simulink model "MicroFSMPCCLACPU1"  (R2024a)
settings: Solver=FixedStepAuto  StartTime=0.0  StopTime=Inf  RelTol=1e-3  EnableMultiTasking=on
values from neighbouring files (symbols this model uses):
  ar = single(round(1/10,3))    [Para_Motor_Micro.m]
  PI_params = mcb.internal.SetControllerParameters(pmsm,inverter,SI_System,T_pwm,Ts,Ts_speed)    [Para_Motor_Micro.m]
  Tabf = round(Tab',3)    [Para_Motor_Micro.m]
  target = mcb_SetProcessorDetails('F28379D',PWM_frequency)    [Para_Motor_Micro.m]
  Ts = T_pwm    (= 3e-05)    [Para_Motor_Micro.m]
  Ts_com = 2*1*Ts    (= 6e-05)    [Para_Motor_Micro.m]
undefined symbols (not defined in the file or in its folder): C28x, codertarget, CPU1, CPU2, Down, dyV, gmax, GPTRIP1SEL, GPTRIP2SEL, inverter, Ls, PWM_Counter_PeriodVel, R, Tab, Tv, Tvz, TZ1, TZ2, ud, Up
libraries: mcbcontrolslib x28, c2802xlib x18, c2837xDlib x13, dsparch4 x6, eeTransforms x5, slpidlib x4, mcbpositiondecoderlib x3, simulink x2, c2806xlib x1, spsabctoAlphaBetaZeroLib x1, c280xlib x1, c2000lib x1
(part 3 of 8)

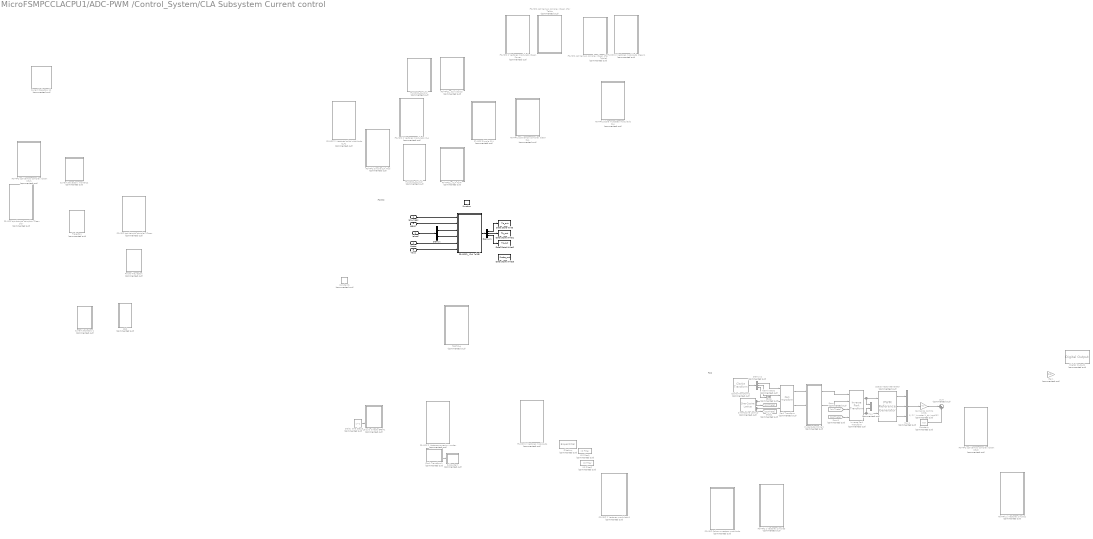
== system MicroFSMPCCLACPU1/ADC-PWM /Control_System/CLA Subsystem Current control ==
  note: FOC
  note: FSMPC
  Iab_meas : Inport
  Iabref : Inport  Port=2
  BEMF : Inport  Port=3
  Moder : Inport  Port=4
  Vbus : Inport  Port=5
  function : TriggerPort  TriggerType=function-call  VariantControl=(inherit)
  Calculo directo BFEM1 : MATLAB Function  Commented=on  TreatAsAtomicUnit=on
  Clark Transform1 : Subsystem  Commented=on
      settings: PortSchema="{\"entries\":[{\"content\":{\"sides\":[{\"content\":{\"connectorIds\":[\"In1\"]},\"type\":\"ConnectorPlacement.EquallySpacedRectSide\",\"uuid\":\"66940a32-98ed-4d42-b87c-a168e8060b1d\"},{\"content\":{\"connectorIds\":[\"Out1\",\"Out2\"],\"side\":\"RIGHT\"},\"type\":\"ConnectorPlacement.EquallySpacedRectSide\",\"uuid\":\"b045ffba-b3d8-4121-bbdc-9875b01ad1c0\"},{\"content\":{\"connectorIds\":[],\"side\":\"TOP\"},\"type\":\"ConnectorPlacement.EquallySpacedRectSide\",\"uuid\":\"4e19d047-7512-4d3b-a0ed-f9cfdeafce15\"},{\"content\":{\"connectorIds\":[\"In2\"],\"side\":\"BOTTOM\"},\"type\":\"ConnectorPlacement.EquallySpacedRectSide\",\"uuid\":\"62e76eb5-f8bd-4841-a5e0-53accc8eabe6\"}]},\"type\":\"ConnectorPlacement.EquallySpacedConnector\",\"uuid\":\"928147e2-84f8-479f-baed-93678fbc2e69\"}],\"packageUris\":[\"http://schema.mathworks.com/mf0/Connector/R2020b\"],\"version\":\"1.0\"}"
  Clarke Transform2 : eeTransforms/Clarke Transform  Commented=on  PowerInvariant=off
  Constant : Constant  Commented=on  Value=0.5  OutDataTypeStr=dataType  SampleTime=-1
  Constant1 : Constant  Commented=on  Value=[0,0,0]  OutDataTypeStr=single
  Current trajectory1 : MATLAB Function  Commented=on  TreatAsAtomicUnit=on
  Current trajectory12 : MATLAB Function  Commented=on  TreatAsAtomicUnit=on
  Current trayectory moder12 : MATLAB Function  Commented=on  TreatAsAtomicUnit=on
  Current_Controllers : Subsystem  Commented=on
  Data Store Write : DataStoreWrite  DataStoreName=Ta_out  IndexOptions=Index vector (dialog)  Indices=1  OutputSizes=1
  Data Store Write1 : DataStoreWrite  DataStoreName=Tb_out  IndexOptions=Index vector (dialog)  Indices=1  OutputSizes=1
  Data Store Write2 : DataStoreWrite  DataStoreName=Tc_out  IndexOptions=Index vector (dialog)  Indices=1  OutputSizes=1
  Data Store Write3 : DataStoreWrite  DataStoreName=Probe_out  IndexOptions=Index vector (dialog)  Indices=1  OutputSizes=1
  Delay One Step3 : Delay  Commented=on  DelayLength=1
  Demux : Demux  Outputs=2
  Demux1 : Demux  Outputs=3
  Demux2 : Demux  Commented=on  Outputs=3
  Digital Output1 : c2837xDlib/Digital Output  Commented=on  GPIO_Number=GPIO32~GPIO39  GPIO_Bit0=off  GPIO_BIT0_Toggle=on  GPIO_Bit1=off  GPIO_BIT1_Toggle=off  GPIO_Bit2=off  GPIO_BIT2_Toggle=off  GPIO_Bit3=off  GPIO_BIT3_Toggle=off  GPIO_Bit4=off  GPIO_BIT4_Toggle=off  GPIO_Bit5=off  GPIO_BIT5_Toggle=off  GPIO_Bit6=off  GPIO_BIT6_Toggle=off  GPIO_Bit7=on  GPIO_BIT7_Toggle=off
  FS-MPC 2 Vectores correcion moder : MATLAB Function  Commented=on  TreatAsAtomicUnit=on
  FS-MPC 2 Vectores modulado : MATLAB Function  Commented=on  TreatAsAtomicUnit=on
  FS-MPC 2 Vectores modulado CLA : MATLAB Function  Commented=on  TreatAsAtomicUnit=on
  FS-MPC 2 Vectores modulado Clean Power : MATLAB Function  Commented=on  TreatAsAtomicUnit=on
  FS-MPC 2 Vectores modulado Clean1 : MATLAB Function  Commented=on  TreatAsAtomicUnit=on
  FS-MPC 2 Vectores modulado1 : MATLAB Function  Commented=on  TreatAsAtomicUnit=on
  FS-MPC 2 Vectores simple2 : MATLAB Function  Commented=on  TreatAsAtomicUnit=on
  FS-MPC 2 Vectores simple3 : MATLAB Function  Commented=on  TreatAsAtomicUnit=on
  FS-MPC 2 Vectores solos modulado CLA1 : MATLAB Function  Commented=on  TreatAsAtomicUnit=on
  FS-MPC Simple CLA : MATLAB Function  Commented=on  TreatAsAtomicUnit=on
  FS-MPC Simple CLA Mod : MATLAB Function  Commented=on  TreatAsAtomicUnit=on
  FS-MPC Sobre muestreo modulado : MATLAB Function  Commented=on  TreatAsAtomicUnit=on
  FS-MPC Sobre muestreo modulado CLA : MATLAB Function  Commented=on  TreatAsAtomicUnit=on
  FS-MPC opt tiempo complex Clean : MATLAB Function  Commented=on  TreatAsAtomicUnit=on
  FS-MPC opt tiempo complex Clean 1for : MATLAB Function  Commented=on  TreatAsAtomicUnit=on
  FS-MPC opt tiempo complex Clean 1for Table : MATLAB Function  Commented=on  TreatAsAtomicUnit=on
  FS-MPC opt tiempo complex Clean 1for Table1 : MATLAB Function  Commented=on  TreatAsAtomicUnit=on
  FS-MPC opt tiempo complex Clean 1for1 : MATLAB Function  Commented=on  TreatAsAtomicUnit=on
  FS-MPC opt tiempo complex Clean 1for2 : MATLAB Function  Commented=on  TreatAsAtomicUnit=on
  FS-MPC opt tiempo complex Clean CLA : MATLAB Function  Commented=on  TreatAsAtomicUnit=on
  FS-MPC1_ CLA 10s(21) : MATLAB Function  Commented=on  TreatAsAtomicUnit=on
  "FS-MPC1_ CLA 4s(9) " : MATLAB Function  Commented=on  TreatAsAtomicUnit=on
  "FS-MPC1_ CLA 7s(15) " : MATLAB Function  TreatAsAtomicUnit=on
  FS-MPC2_CLA(10) : MATLAB Function  Commented=on  TreatAsAtomicUnit=on
  FS-MPC2_CLA(21) : MATLAB Function  Commented=on  TreatAsAtomicUnit=on
  Filterlow : dsparch4/Biquad Filter  Tag=BlockMethodSubSystem  Commented=on  FilterSource=Dialog parameters  CoeffSource=Specify via dialog  FilterObject=BQF  IIRFiltStruct=Direct form II  BiQuadCoeffs=[1 1 0 1 0.350634150167160374 0]  ScaleValues=[0.675317075083580187;1]  IC=0  ICnum=0  ICden=0  a0Flag=Warning  optimizeScaleValues=on  ScaleValueMode=Specify via input port (g)  InputProcessing=Columns as channels (frame based)  roundingMode=Floor  overflowMode=off  scaleValueFracLength=14  denProdOutputFracLength=30  denAccumFracLength=30  secondMemoryFracLength=15
  From : From  Commented=on  GotoTag=sinTheta
  From1 : From  Commented=on  GotoTag=cosTheta
  Gain : Gain  Commented=on  Gain=0.9  OutDataTypeStr=single
  Goto : Goto  Commented=on  GotoTag=sinTheta
  Goto1 : Goto  Commented=on  GotoTag=cosTheta
  IIR Filter1 : mcbcontrolslib/IIR Filter  Commented=on  VariantControl=Low Pass Filter  VariantSelect=Low-pass  FilterConstantInputType=Specify via dialog  Filter_constant=0.3  advancedSettings=off  Ts=5e-5  cutOff_freq=1364.1852
  IIR Filter2 : mcbcontrolslib/IIR Filter  Commented=on  VariantControl=Low Pass Filter  VariantSelect=Low-pass  FilterConstantInputType=Specify via dialog  Filter_constant=0.3  advancedSettings=off  Ts=5e-5  cutOff_freq=1364.1852
  Inverse Park Transform : mcbcontrolslib/Inverse Park Transform  Commented=on  PhaseInput=Two inputs  AxisAlignment=D-axis  ThetaInput=Sine and Cosine electrical position  AngleInput=Per-unit  N_points=1024
  Mux : Mux  Commented=on  Inputs=2
  Mux1 : Mux  Commented=on  Inputs=3
  Normalize [-0.5 to 0.5]1 : Gain  Commented=on  Gain=1/ (2 * inverter.V_dc / sqrt(3))  RndMeth=Simplest  OutDataTypeStr=Inherit: Same as input
  Park Transform : mcbcontrolslib/Park Transform  Commented=on  PhaseInput=Two inputs  AxisAlignment=D-axis  ThetaInput=Sine and Cosine electrical position  AngleInput=Per-unit  N_points=1024
  Power Trayectory : MATLAB Function  Commented=on  TreatAsAtomicUnit=on
  Sine-Cosine Lookup : mcbcontrolslib/Sine-Cosine Lookup  Commented=on  AngleInput=Radians  N_points=1024  DatatypeInput=Inherit from input  Datatype=single
  Space Vector Generator : mcbcontrolslib/PWM Reference Generator  Commented=on  inSignal=Valphabeta  modType=SVM: space vector modulation
  Subsystem : Subsystem  Commented=on
  Sum : Sum  Commented=on  Inputs=|++
  TESTCLA : MATLAB Function  Commented=on
  Terminator2 : Terminator  Commented=on
  Trajectory : MATLAB Function  Commented=on  TreatAsAtomicUnit=on
  stp2 : MATLAB Function  Commented=on  TreatAsAtomicUnit=on
  wires:
  Demux/1 -> "FS-MPC1_ CLA 7s(15) "/3(iAref)
  Clark Transform1/2(Fcemab) -> Subsystem/1(FCEM)
  Current_Controllers/1(Vd_ref) -> Inverse Park Transform/1
  Delay One Step3/1 -> Calculo directo BFEM1/3(Iant)
  Park Transform/2 -> Current_Controllers/2(Iq)
  From/1 -> Inverse Park Transform/3
  Demux/2 -> "FS-MPC1_ CLA 7s(15) "/4(iBref)
  From1/1 -> Inverse Park Transform/4
  Inverse Park Transform/1 -> Mux/1, Space Vector Generator/1
  Park Transform/1 -> Current_Controllers/1(Id)
  Normalize [-0.5 to 0.5]1/1 -> Sum/1
  Space Vector Generator/3 -> Mux1/3
  Current_Controllers/2(Vq_ref) -> Inverse Park Transform/2
  Clarke Transform2/1 -> Demux2/1
  Constant/1 -> Sum/2
  Demux2/1 -> Park Transform/1
  Iabref/1 -> Demux/1
  Mux1/1 -> Normalize [-0.5 to 0.5]1/1
  Space Vector Generator/2 -> Mux1/2
  Space Vector Generator/1 -> Mux1/1
  Demux2/3 -> Terminator2/1
  Moder/1 -> "FS-MPC1_ CLA 7s(15) "/5(mode)
  Demux2/2 -> Park Transform/2
  Sine-Cosine Lookup/2 -> Park Transform/4, Goto1/1
  Sine-Cosine Lookup/1 -> Goto/1, Park Transform/3
  Inverse Park Transform/2 -> Space Vector Generator/2, Mux/2
  Demux1/1 -> Data Store Write/1
  Demux1/2 -> Data Store Write1/1
  Demux1/3 -> Data Store Write2/1
  BEMF/1 -> "FS-MPC1_ CLA 7s(15) "/2(FEM)
  Vbus/1 -> "FS-MPC1_ CLA 7s(15) "/6(ud)
  "FS-MPC1_ CLA 7s(15) "/1(Gate) -> Demux1/1
  Iab_meas/1 -> "FS-MPC1_ CLA 7s(15) "/1(I)

== system MicroFSMPCCLACPU1/ADC-PWM /Control_System/Clark Transform Filter ==
  Iabc : Inport
  Clarke Transformation : Subsystem  InitFcn=tic2000lib_licenseCheck  mask(Clarke Transformation){}
      mask help: This block performs transformation of three-phase quantities into balanced two-phase quadrature quantities. All inputs and outputs are signed 32-bit fixed-point numbers with Q value between 1 and 29.
      mask Help: eval('linkfoundation.util.openBlockHelp(''c28xdmclibclarketransformation'',''ecoder'')');
      mask Display:
      | port_label('input',1,'As');
      | port_label('input',2,'Bs');
      | port_label('Output',1,'Alpha');
      | port_label('Output',2,'Beta');
      | text(0.5,0.15, 'Clarke', 'horizontalalignment','center');
  Demux : Demux  Outputs=3
  Mux1 : Mux  Inputs=2
  Iab : Outport
  wires:
  Iabc/1 -> Demux/1
  Clarke Transformation/1(Out1) -> Mux1/1
  Clarke Transformation/2(Out2) -> Mux1/2
  Demux/2 -> Clarke Transformation/2(Ib)
  Demux/1 -> Clarke Transformation/1(Ia)
  Mux1/1 -> Iab/1

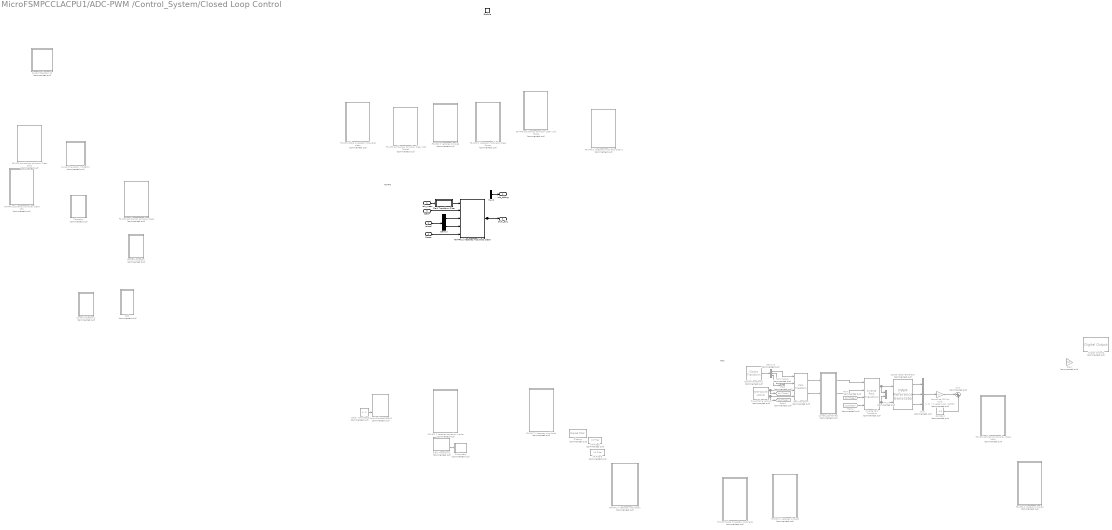
== system MicroFSMPCCLACPU1/ADC-PWM /Control_System/Closed Loop Control ==
  note: FSMPC
  note: FOC
  Iab_meas : Inport
  Iabref : Inport  Port=2
  BEMF : Inport  Port=3
  Moder : Inport  Port=4
  Enable : EnablePort  StatesWhenEnabling=reset
  Calculo directo BFEM1 : MATLAB Function  Commented=on  TreatAsAtomicUnit=on
  Clark Transform Filter : Subsystem
  Clark Transform1 : Subsystem  Commented=on
      settings: PortSchema="{\"entries\":[{\"content\":{\"sides\":[{\"content\":{\"connectorIds\":[\"In1\"]},\"type\":\"ConnectorPlacement.EquallySpacedRectSide\",\"uuid\":\"66940a32-98ed-4d42-b87c-a168e8060b1d\"},{\"content\":{\"connectorIds\":[\"Out1\",\"Out2\"],\"side\":\"RIGHT\"},\"type\":\"ConnectorPlacement.EquallySpacedRectSide\",\"uuid\":\"b045ffba-b3d8-4121-bbdc-9875b01ad1c0\"},{\"content\":{\"connectorIds\":[],\"side\":\"TOP\"},\"type\":\"ConnectorPlacement.EquallySpacedRectSide\",\"uuid\":\"4e19d047-7512-4d3b-a0ed-f9cfdeafce15\"},{\"content\":{\"connectorIds\":[\"In2\"],\"side\":\"BOTTOM\"},\"type\":\"ConnectorPlacement.EquallySpacedRectSide\",\"uuid\":\"62e76eb5-f8bd-4841-a5e0-53accc8eabe6\"}]},\"type\":\"ConnectorPlacement.EquallySpacedConnector\",\"uuid\":\"928147e2-84f8-479f-baed-93678fbc2e69\"}],\"packageUris\":[\"http://schema.mathworks.com/mf0/Connector/R2020b\"],\"version\":\"1.0\"}"
  Clarke Transform2 : eeTransforms/Clarke Transform  Commented=on  PowerInvariant=off
  Constant : Constant  Commented=on  Value=0.5  OutDataTypeStr=dataType  SampleTime=-1
  Current trajectory1 : MATLAB Function  Commented=on  TreatAsAtomicUnit=on
  Current trajectory12 : MATLAB Function  Commented=on  TreatAsAtomicUnit=on
  Current trayectory moder12 : MATLAB Function  Commented=on  TreatAsAtomicUnit=on
  Current_Controllers : Subsystem  Commented=on
  Delay One Step3 : Delay  Commented=on  DelayLength=1
  Demux : Demux  Outputs=2
  Demux2 : Demux  Commented=on  Outputs=3
  Digital Output1 : c2837xDlib/Digital Output  Commented=on  GPIO_Number=GPIO32~GPIO39  GPIO_Bit0=off  GPIO_BIT0_Toggle=on  GPIO_Bit1=off  GPIO_BIT1_Toggle=off  GPIO_Bit2=off  GPIO_BIT2_Toggle=off  GPIO_Bit3=off  GPIO_BIT3_Toggle=off  GPIO_Bit4=off  GPIO_BIT4_Toggle=off  GPIO_Bit5=off  GPIO_BIT5_Toggle=off  GPIO_Bit6=off  GPIO_BIT6_Toggle=off  GPIO_Bit7=on  GPIO_BIT7_Toggle=off
  FS-MPC 2 Vectores correcion moder : MATLAB Function  Commented=on  TreatAsAtomicUnit=on
  FS-MPC 2 Vectores modulado : MATLAB Function  Commented=on  TreatAsAtomicUnit=on
  FS-MPC 2 Vectores modulado Clean : MATLAB Function  TreatAsAtomicUnit=on
  FS-MPC 2 Vectores modulado Clean Power : MATLAB Function  Commented=on  TreatAsAtomicUnit=on
  FS-MPC 2 Vectores modulado Clean1 : MATLAB Function  Commented=on  TreatAsAtomicUnit=on
  FS-MPC 2 Vectores modulado1 : MATLAB Function  Commented=on  TreatAsAtomicUnit=on
  FS-MPC 2 Vectores simple1 : MATLAB Function  Commented=on  TreatAsAtomicUnit=on
  FS-MPC 2 Vectores simple2 : MATLAB Function  Commented=on  TreatAsAtomicUnit=on
  FS-MPC 2 Vectores simple3 : MATLAB Function  Commented=on  TreatAsAtomicUnit=on
  FS-MPC Sobre muestreo modulado : MATLAB Function  Commented=on  TreatAsAtomicUnit=on
  FS-MPC Sobre muestreo modulado clean : MATLAB Function  Commented=on  TreatAsAtomicUnit=on
  FS-MPC opt tiempo complex Clean : MATLAB Function  Commented=on  TreatAsAtomicUnit=on
  FS-MPC opt tiempo complex Clean 1for : MATLAB Function  Commented=on  TreatAsAtomicUnit=on
  FS-MPC opt tiempo complex Clean 1for Table : MATLAB Function  Commented=on  TreatAsAtomicUnit=on
  FS-MPC opt tiempo complex Clean 1for Table1 : MATLAB Function  Commented=on  TreatAsAtomicUnit=on
  FS-MPC opt tiempo complex Clean 1for1 : MATLAB Function  Commented=on  TreatAsAtomicUnit=on
  FS-MPC opt tiempo complex Clean 1for2 : MATLAB Function  Commented=on  TreatAsAtomicUnit=on
  Filterlow : dsparch4/Biquad Filter  Tag=BlockMethodSubSystem  Commented=on  FilterSource=Dialog parameters  CoeffSource=Specify via dialog  FilterObject=BQF  IIRFiltStruct=Direct form II  BiQuadCoeffs=[1 1 0 1 0.350634150167160374 0]  ScaleValues=[0.675317075083580187;1]  IC=0  ICnum=0  ICden=0  a0Flag=Warning  optimizeScaleValues=on  ScaleValueMode=Specify via input port (g)  InputProcessing=Columns as channels (frame based)  roundingMode=Floor  overflowMode=off  scaleValueFracLength=14  denProdOutputFracLength=30  denAccumFracLength=30  secondMemoryFracLength=15
  From : From  Commented=on  GotoTag=sinTheta
  From1 : From  Commented=on  GotoTag=cosTheta
  Gain : Gain  Commented=on  Gain=0.9  OutDataTypeStr=single
  Goto : Goto  Commented=on  GotoTag=sinTheta
  Goto1 : Goto  Commented=on  GotoTag=cosTheta
  IIR Filter1 : mcbcontrolslib/IIR Filter  Commented=on  VariantControl=Low Pass Filter  VariantSelect=Low-pass  FilterConstantInputType=Specify via dialog  Filter_constant=0.3  advancedSettings=off  Ts=5e-5  cutOff_freq=1364.1852
  IIR Filter2 : mcbcontrolslib/IIR Filter  Commented=on  VariantControl=Low Pass Filter  VariantSelect=Low-pass  FilterConstantInputType=Specify via dialog  Filter_constant=0.3  advancedSettings=off  Ts=5e-5  cutOff_freq=1364.1852
  Inverse Park Transform : mcbcontrolslib/Inverse Park Transform  Commented=on  PhaseInput=Two inputs  AxisAlignment=D-axis  ThetaInput=Sine and Cosine electrical position  AngleInput=Per-unit  N_points=1024
  Mux : Mux  Commented=on  Inputs=2
  Mux1 : Mux  Commented=on  Inputs=3
  Mux2 : Mux  Inputs=2
  Normalize [-0.5 to 0.5]1 : Gain  Commented=on  Gain=1/ (2 * inverter.V_dc / sqrt(3))  RndMeth=Simplest  OutDataTypeStr=Inherit: Same as input
  Park Transform : mcbcontrolslib/Park Transform  Commented=on  PhaseInput=Two inputs  AxisAlignment=D-axis  ThetaInput=Sine and Cosine electrical position  AngleInput=Per-unit  N_points=1024
  Power Trayectory : MATLAB Function  Commented=on  TreatAsAtomicUnit=on
  Sine-Cosine Lookup : mcbcontrolslib/Sine-Cosine Lookup  Commented=on  AngleInput=Radians  N_points=1024  DatatypeInput=Inherit from input  Datatype=single
  Space Vector Generator : mcbcontrolslib/PWM Reference Generator  Commented=on  inSignal=Valphabeta  modType=SVM: space vector modulation
  Subsystem : Subsystem  Commented=on
  Sum : Sum  Commented=on  Inputs=|++
  Terminator2 : Terminator  Commented=on
  Trajectory : MATLAB Function  Commented=on  TreatAsAtomicUnit=on
  stp2 : MATLAB Function  Commented=on  TreatAsAtomicUnit=on
  Idq_debug : Outport  VectorParamsAs1DForOutWhenUnconnected=off
  Duty_abc : Outport  Port=2  VectorParamsAs1DForOutWhenUnconnected=off
  wires:
  Park Transform/1 -> Current_Controllers/1(Id)
  Sine-Cosine Lookup/2 -> Park Transform/4, Goto1/1
  Sine-Cosine Lookup/1 -> Goto/1, Park Transform/3
  Demux2/2 -> Park Transform/2
  From1/1 -> Inverse Park Transform/4
  From/1 -> Inverse Park Transform/3
  Current_Controllers/1(Vd_ref) -> Inverse Park Transform/1
  Current_Controllers/2(Vq_ref) -> Inverse Park Transform/2
  Inverse Park Transform/1 -> Mux/1, Space Vector Generator/1
  Inverse Park Transform/2 -> Space Vector Generator/2, Mux/2
  Space Vector Generator/3 -> Mux1/3
  Space Vector Generator/2 -> Mux1/2
  Space Vector Generator/1 -> Mux1/1
  Normalize [-0.5 to 0.5]1/1 -> Sum/1
  Mux1/1 -> Normalize [-0.5 to 0.5]1/1
  Constant/1 -> Sum/2
  Park Transform/2 -> Current_Controllers/2(Iq)
  Demux2/3 -> Terminator2/1
  Clarke Transform2/1 -> Demux2/1
  Delay One Step3/1 -> Calculo directo BFEM1/3(Iant)
  Iab_meas/1 -> Clark Transform Filter/1(Iabc)
  Clark Transform Filter/1(Iab) -> FS-MPC 2 Vectores modulado Clean/1(I)
  Clark Transform1/2(Fcemab) -> Subsystem/1(FCEM)
  Mux2/1 -> Idq_debug/1
  Demux2/1 -> Park Transform/1
  Iabref/1 -> Demux/1
  BEMF/1 -> FS-MPC 2 Vectores modulado Clean/2(FEM)
  FS-MPC 2 Vectores modulado Clean/1(Gate) -> Duty_abc/1
  Demux/1 -> FS-MPC 2 Vectores modulado Clean/3(iAref)
  Demux/2 -> FS-MPC 2 Vectores modulado Clean/4(iBref)
  Moder/1 -> FS-MPC 2 Vectores modulado Clean/5(mode)

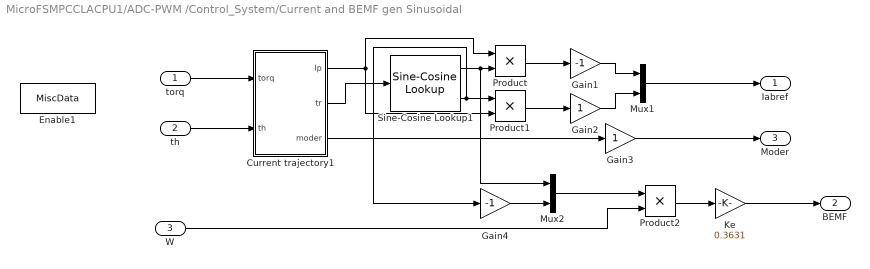
== system MicroFSMPCCLACPU1/ADC-PWM /Control_System/Current and BEMF gen Sinusoidal ==
  torq : Inport
  th : Inport  Port=2
  W : Inport  Port=3
  Current trajectory1 : MATLAB Function  TreatAsAtomicUnit=on
  Enable1 : DataStoreRead  DataStoreName=MiscData  IndexOptions=Index vector (dialog)  Indices=1  OutputSizes=1
  Gain1 : Gain  Gain=-1  OutDataTypeStr=single
  Gain2 : Gain  OutDataTypeStr=single
  Gain3 : Gain  OutDataTypeStr=single
  Gain4 : Gain  Gain=-1  OutDataTypeStr=single
  Ke : Gain  Gain=0.3631  OutDataTypeStr=single
  Mux1 : Mux  Inputs=2
  Mux2 : Mux  Inputs=2
  Product : Product  OutDataTypeStr=single
  Product1 : Product  OutDataTypeStr=single
  Product2 : Product  OutDataTypeStr=single
  Sine-Cosine Lookup1 : mcbcontrolslib/Sine-Cosine Lookup  AngleInput=Radians  N_points=1024  DatatypeInput=Specify via dialog  Datatype=single
  Iabref : Outport
  BEMF : Outport  Port=2
  Moder : Outport  Port=3
  wires:
  Current trajectory1/1(Ip) -> Product/1, Product1/2
  Mux2/1 -> Product2/1
  Sine-Cosine Lookup1/2 -> Gain4/1, Product1/1
  Product1/1 -> Gain2/1
  Product/1 -> Gain1/1
  torq/1 -> Current trajectory1/1(torq)
  W/1 -> Product2/2
  Product2/1 -> Ke/1
  Sine-Cosine Lookup1/1 -> Mux2/1, Product/2
  th/1 -> Current trajectory1/2(th)
  Current trajectory1/3(moder) -> Gain3/1
  Ke/1 -> BEMF/1
  Gain1/1 -> Mux1/1
  Gain2/1 -> Mux1/2
  Mux1/1 -> Iabref/1
  Gain3/1 -> Moder/1
  Gain4/1 -> Mux2/2
  Current trajectory1/2(tr) -> Sine-Cosine Lookup1/1

== system MicroFSMPCCLACPU1/ADC-PWM /Control_System/Current and BEMF gen Trapezoidal ==
  torq : Inport
  th : Inport  Port=2
  W : Inport  Port=3
  Current trajectory2 : MATLAB Function  TreatAsAtomicUnit=on
  Enable1 : DataStoreRead  DataStoreName=MiscData  IndexOptions=Index vector (dialog)  Indices=1  OutputSizes=1
  Mux : Mux  Inputs=2
  Iabref : Outport
  BEMF : Outport  Port=2
  Moder : Outport  Port=3
  wires:
  Current trajectory2/4(eab) -> BEMF/1
  th/1 -> Current trajectory2/2(th)
  torq/1 -> Current trajectory2/1(torq)
  W/1 -> Current trajectory2/3(w)
  Current trajectory2/2(Ib) -> Mux/2
  Current trajectory2/1(Ia) -> Mux/1
  Mux/1 -> Iabref/1
  Current trajectory2/3(moder) -> Moder/1

== system MicroFSMPCCLACPU1/ADC-PWM /Control_System/Te_calculation ==
  Iab : Inport
  Omega : Inport  Port=2
  FCEM : Inport  Port=3
  Add : Sum  Commented=on
  Demux : Demux  Commented=on  Outputs=2
  Demux1 : Demux  Commented=on  Outputs=2
  Divide : Product  Commented=on  Inputs=*/
  Gain : Gain  Commented=on  Gain=-1
  Product : Product  Commented=on
  Product1 : Product  Commented=on
  Te : Outport
  wires:
  Add/1 -> Divide/1
  Gain/1 -> Demux/1
  Demux/1 -> Product/1
  Demux1/2 -> Product1/2
  Product/1 -> Add/1
  Product1/1 -> Add/2
  FCEM/1 -> Gain/1
  Demux1/1 -> Product/2
  Omega/1 -> Divide/2
  Demux/2 -> Product1/1
  Iab/1 -> Demux1/1
  Divide/1 -> Te/1

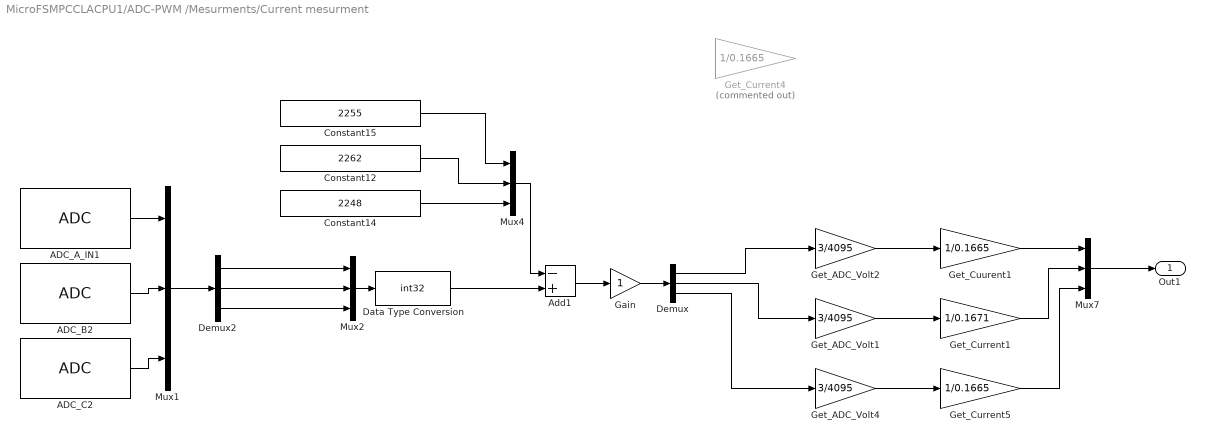
== system MicroFSMPCCLACPU1/ADC-PWM /Mesurments/Current mesurment ==
  ADC_A_IN1 : c2802xlib/ADC  blkParamProc=C2000_Type4  ADCModule=B  samplingMode=Single sample mode  ADCResolution=12-bit (Single-ended input)  useSOC1=SOC0  useSOC2=SOC0_SOC1  SOCAcquisitionWindow=15  SOCTriggerSource=ePWM1_ADCSOCA  SOCInterruptTrigger=No ADCINT  Ts=-1  dType=uint16  postInterrupt=off  interruptSel=ADCINT1  ADCINTContinuous=on  endma=off  chdma=1  conv1=ADCINA0  conv2=ADCINA0 and ADCINB0  conv1_Type4=ADCIN3  conv2_Type4=ADCIN0 and ADCIN1
  ADC_B2 : c2802xlib/ADC  blkParamProc=C2000_Type4  ADCModule=B  samplingMode=Single sample mode  ADCResolution=12-bit (Single-ended input)  useSOC1=SOC1  useSOC2=SOC0_SOC1  SOCAcquisitionWindow=15  SOCTriggerSource=ePWM1_ADCSOCA  SOCInterruptTrigger=No ADCINT  Ts=-1  dType=uint16  postInterrupt=off  interruptSel=ADCINT1  ADCINTContinuous=on  endma=off  chdma=1  conv1=ADCINA0  conv2=ADCINA0 and ADCINB0  conv1_Type4=ADCIN5  conv2_Type4=ADCIN0 and ADCIN1
  ADC_C2 : c2802xlib/ADC  blkParamProc=C2000_Type4  ADCModule=A  samplingMode=Single sample mode  ADCResolution=12-bit (Single-ended input)  useSOC1=SOC0  useSOC2=SOC0_SOC1  SOCAcquisitionWindow=15  SOCTriggerSource=ePWM1_ADCSOCA  SOCInterruptTrigger=No ADCINT  Ts=-1  dType=uint16  postInterrupt=on  interruptSel=ADCINT1  ADCINTContinuous=on  endma=off  chdma=1  conv1=ADCINA0  conv2=ADCINA0 and ADCINB0  conv1_Type4=ADCIN5  conv2_Type4=ADCIN0 and ADCIN1
  Add1 : Sum  Inputs=-+
  Constant12 : Constant  Value=2262  OutDataTypeStr=single
  Constant14 : Constant  Value=2248  OutDataTypeStr=single
  Constant15 : Constant  Value=2255  OutDataTypeStr=single
  Data Type Conversion : DataTypeConversion  OutDataTypeStr=int32  ConvertRealWorld=Stored Integer (SI)  RndMeth=Simplest  SaturateOnIntegerOverflow=off
  Demux : Demux  Outputs=3
  Demux2 : Demux  Outputs=3
  Gain : Gain  OutDataTypeStr=single
  Get_ADC_Volt1 : Gain  Gain=3/4095  OutDataTypeStr=single  RndMeth=Simplest
  Get_ADC_Volt2 : Gain  Gain=3/4095  OutDataTypeStr=single  RndMeth=Simplest
  Get_ADC_Volt4 : Gain  Gain=3/4095  OutDataTypeStr=single  RndMeth=Simplest
  Get_Current1 : Gain  Gain=1/0.1671  OutDataTypeStr=single  RndMeth=Simplest
  Get_Current4 : Gain  Commented=on  Gain=1/0.1665  OutDataTypeStr=single  RndMeth=Simplest
  Get_Current5 : Gain  Gain=1/0.1665  OutDataTypeStr=single  RndMeth=Simplest
  Get_Cuurent1 : Gain  Gain=1/0.1665  OutDataTypeStr=single  RndMeth=Simplest
  Mux{1..2,4,7} (4 alike) : Mux  Inputs=3
  Out1 : Outport
  wires:
  Data Type Conversion/1 -> Add1/2
  ADC_C2/1 -> Mux1/3
  Mux2/1 -> Data Type Conversion/1
  Demux2/2 -> Mux2/2
  Add1/1 -> Gain/1
  Demux2/3 -> Mux2/3
  Mux1/1 -> Demux2/1
  Mux4/1 -> Add1/1
  Demux/1 -> Get_ADC_Volt2/1
  ADC_B2/1 -> Mux1/2
  Constant12/1 -> Mux4/2
  Demux/2 -> Get_ADC_Volt1/1
  Get_ADC_Volt2/1 -> Get_Cuurent1/1
  ADC_A_IN1/1 -> Mux1/1
  Get_ADC_Volt4/1 -> Get_Current5/1
  Get_ADC_Volt1/1 -> Get_Current1/1
  Constant15/1 -> Mux4/1
  Demux/3 -> Get_ADC_Volt4/1
  Constant14/1 -> Mux4/3
  Demux2/1 -> Mux2/1
  Mux7/1 -> Out1/1
  Get_Cuurent1/1 -> Mux7/1
  Get_Current1/1 -> Mux7/2
  Get_Current5/1 -> Mux7/3
  Gain/1 -> Demux/1

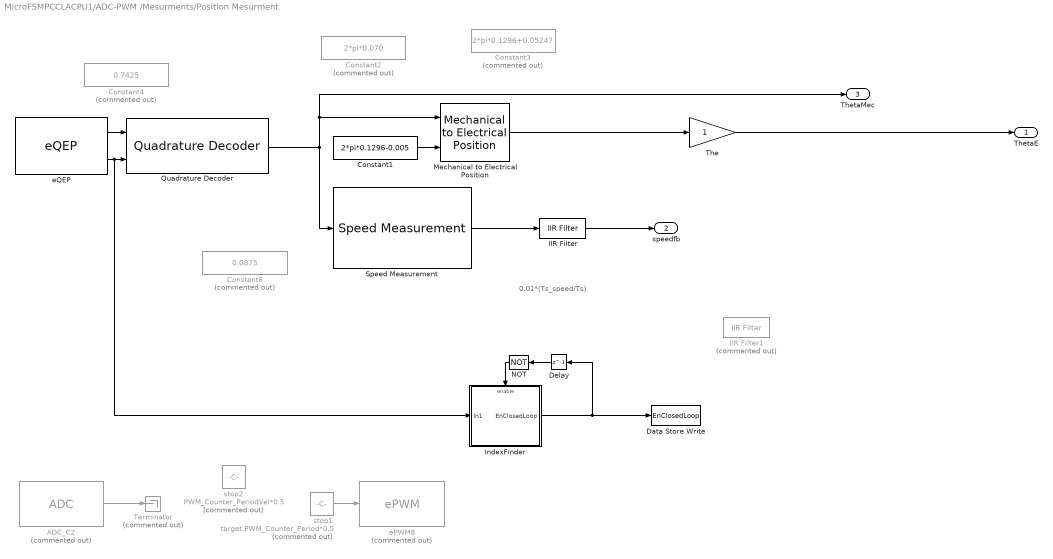
== system MicroFSMPCCLACPU1/ADC-PWM /Mesurments/Position Mesurment ==
  note: 0.01*(Ts_speed/Ts)
  ADC_C2 : c2802xlib/ADC  Commented=on  blkParamProc=C2000_Type4  ADCModule=C  samplingMode=Single sample mode  ADCResolution=12-bit (Single-ended input)  useSOC1=SOC5  useSOC2=SOC0_SOC1  SOCAcquisitionWindow=15  SOCTriggerSource=ePWM4_ADCSOCA  SOCInterruptTrigger=No ADCINT  Ts=-1  dType=uint16  postInterrupt=on  interruptSel=ADCINT1  ADCINTContinuous=on  endma=off  chdma=1  conv1=ADCINA0  conv2=ADCINA0 and ADCINB0  conv1_Type4=ADCIN0  conv2_Type4=ADCIN0 and ADCIN1
  Constant1 : Constant  Value=2*pi*0.1296-0.005  OutDataTypeStr=single
  Constant2 : Constant  Commented=on  Value=2*pi*0.070  OutDataTypeStr=single
  Constant3 : Constant  Commented=on  Value=2*pi*0.1296+0.05247  OutDataTypeStr=single
  Constant4 : Constant  Commented=on  Value=0.7425  OutDataTypeStr=single
  Constant6 : Constant  Commented=on  Value=0.0875  OutDataTypeStr=single
  Data Store Write : DataStoreWrite  DataStoreName=EnClosedLoop  IndexOptions=Index vector (dialog)  Indices=1  OutputSizes=1
  Delay : Delay  DelayLength=1
  IIR Filter : mcbcontrolslib/IIR Filter  VariantControl=Low Pass Filter  VariantSelect=Low-pass  FilterConstantInputType=Specify via dialog  Filter_constant=0.01  advancedSettings=off  Ts=10e-6  cutOff_freq=160.7626
  IIR Filter1 : mcbcontrolslib/IIR Filter  Commented=on  VariantControl=Low Pass Filter  VariantSelect=Low-pass  FilterConstantInputType=Specify via dialog  Filter_constant=0.0095  advancedSettings=off  Ts=10e-6  cutOff_freq=152.6473
  IndexFinder : Subsystem
  Mechanical to Electrical Position : mcbpositiondecoderlib/Mechanical to Electrical Position  PolePairsInputType=Specify via dialog  NrPP=4  selectedRange=Radians  MechOfstInputType=Input port  mechOffsetIn=0  maxAngleIn=2*pi  InputDataType=single  VariantSelect=floating-point
  NOT : Logic  Operator=NOT  AllPortsSameDT=off  OutDataTypeStr=boolean
  Quadrature Decoder : mcbpositiondecoderlib/Quadrature Decoder  EncoderSlitsPerRevolution=2048  EncoderCountsPerSlit=4  CounterSize=16 bits  ExternalIndexCount=on  PositionUnit=Radians  PositionDataType=single  ParameterInputType=off  CountsPerRevInverseDataType=single
  Speed Measurement : mcbpositiondecoderlib/Speed Measurement  PositionUnit=Radians  PositionScalingDatatype=uint32  SpeedCalculationMode=Time interval for speed calculation  SampleTimeAsync=Ts  MaximumApplicationSpeed=6000  SpeedResolution=5e-6  DelayLength=20  MaximumMeasurableSpeed=-0.98352  MeasurableSpeedResolution=7.6757e-12  SpeedUnit=Radians/Sec  PerUnitSpeed=PU_System.N_base  SpeedDataType=single
  Terminator : Terminator  Commented=on
  The : Gain  OutDataTypeStr=single  RndMeth=Simplest
  ePWM8 : c2802xlib/ePWM  Commented=on  PwmType=C2000_Type4  useModule=ePWM4  ePWMxLINKTBPRD=Not Linked  periodUnits=Clock cycles  timerSource=Specify via dialog  timerPeriod_clk=PWM_Counter_PeriodVel+1  timerPeriod_sec=0.0001  tbshadow=Counter equals to zero  countingMode=Up-Down  phaseActiveEnable=Disable  phaseDirection=Count down after sync  phaseActive=0  synchronizationEnable=off  dcaevt1Sync=off  dcbevt1Sync=off  synchronizationOption=Counter equals to zero (CTR=Zero)  dcbevt1SyncOut=off  dcaevt1SyncOut=off  cmpdSyncOut=off  cmpcSyncOut=off  cmpbSyncOut=off  zeroSyncOut=on  swfSyncOut=off  perSynchronizationOption=Counter equals to period (CTR=PRD)  clockPrescale=1  HSclockPrescale=1  enswap=off  ePWMxAStatus=on  ePWMxAactionLogic1=Do nothing  ePWMxAactionLogic2=Do nothing  ePWMxAactionLogic3=Clear  ePWMxAactionLogic4=Set  ePWMxAactionLogic5=Do nothing  ePWMxAactionLogic6=Do nothing  ePWMxACSFenable=off  ePWMxACSFvalue=Forcing disable  ePWMxASFreload=Zero  ePWMxBStatus=off  ePWMxBactionLogic1=Set  ePWMxBactionLogic2=Clear  ePWMxBactionLogic3=Do nothing  ePWMxBactionLogic4=Do nothing  ePWMxBactionLogic5=Clear  ePWMxBactionLogic6=Set  ePWMxBCSFenable=off  ePWMxBCSFvalue=Forcing disable  ePWMxBSFreload=Zero  ePWNxBOutWay=off  ePWMxLINKCMPA=Not Linked  CMPAUnits=Clock cycles  CMPASource=Input port  CMPAValue_per=50  CMPAValue_clk=floor(PWM_Counter_PeriodVel/2+1)  enCMPAshadow=Counter equals to zero (CTR=Zero)  ePWMxLINKCMPB=Not Linked  CMPBUnits=Clock cycles  CMPBSource=Specify via dialog  CMPBValue_per=50  CMPBValue_clk=floor(PWM_Counter_PeriodVel/2+1)  enCMPBshadow=Counter equals to zero (CTR=Zero)  ePWMxLINKCMPC=Not Linked  CMPCUnits=Clock cycles  CMPCSource=Specify via dialog  CMPCValue_per=50  CMPCValue_clk=32000  enCMPCshadow=Counter equals to zero (CTR=Zero)  ePWMxLINKCMPD=Not Linked  CMPDUnits=Clock cycles  CMPDSource=Specify via dialog  CMPDValue_per=50  CMPDValue_clk=32000  enCMPDshadow=Counter equals to zero (CTR=Zero)  enableDBePWMxA=on  enableDBePWMxB=on  enhalfcycle=off  DBpolarity=Active high complementary (AHC)  DBedgeDelay=Positive  DBSource_ePWMxA=ePWMxA  DBSource_ePWMxB=ePWMxA  DBPeriodUnits=Clock cycles  DBperiodSource=Specify via dialog  REDperiod=15  FEDperiod=15  REDperiod_sec=0  FEDperiod_sec=0  LoadModeDBRED=Immediate without using shadow  LoadModeDBFED=Immediate without using shadow  adcstartModuleA=on  adcrequestEventA=First event  adcstartEventA=Digital Compare Module A Event 1 start of conversion (DCAEVT1.soc)  adcstartEventA_type2=Counter equals to period (CTR=PRD)  adcstartModuleB=off  adcrequestEventB=First event  adcstartEventB=Counter equals to zero (CTR=Zero)  adcstartEventB_type2=Counter equals to zero (CTR=Zero)  intEn=off  intPrd=First event  intSel=Counter equals to zero (CTR=Zero)  intSel_type2=Counter equals to zero (CTR=Zero)  hrpe=off  enHRPWM=off  HRPWM_LoadMode=Counter equals to period (CTR=PRD)  HRPWM_CTLMode=Duty or Period control mode  HRPWM_EDGMode=Both edge  hrpeb=off  enHRPWMB=off  HRPWM_LoadModeB=Counter equals to zero (CTR=ZERO)  HRPWM_CTLModeB=Duty or Period control mode  HRPWM_EDGModeB=Both edge  enHRDBRED=off  enHRDBFED=off  enSFO=on  enautoconv=on  chopperEnable=off  chopperFrequency=1  chopperFirstwidth=1  chopperDuty=12.5%  tripZonesource=Specify via dialog  tzselOSHT1=off  tzselOSHT2=off  tzselOSHT3=off  tzselOSHT4=off  tzselOSHT5=off  tzselOSHT6=off  tzselOSHDCAEV1=off  tzselOSHDCBEV1=off  tzselCBC1=off  tzselCBC2=off  tzselCBC3=off  tzselCBC4=off  tzselCBC5=off  tzselCBC6=off  tzselCBCDCAEV2=off  tzselCBCDCBEV2=off  enTzOstIntr=off  enTzCbcIntr=off  enTzDCAEVT1Intr=off  enTzDCAEVT2Intr=off  enTzDCBEVT1Intr=off  enTzDCBEVT2Intr=off  tzclrCBCLatch=Counter equals to zero (CTR=Zero)  ePWMxAforced=No action  ePWMxBforced=No action  DCAEVT1forced=No action  DCBEVT1forced=No action  DCAEVT2forced=No action  DCBEVT2forced=No action  dcah=Trip Zone 1 input (TZ1)  dcal=Trip Zone 2 input (TZ2)  dcbh=Trip Zone 1 input (TZ1)  dcbl=Trip Zone 2 input (TZ2)  dcah_type2=GPTRIP1SEL/(TZ1)  dcal_type2=GPTRIP2SEL/(TZ2)  dcbh_type2=GPTRIP1SEL/(TZ1)  dcbl_type2=GPTRIP2SEL/(TZ2)  gendcaevt1=Event disabled  gendcaevt2=Event disabled  gendcbevt1=Event disabled  gendcbevt2=Event disabled  dcaevt1src=DCAEVT1 with sync  dcaevt2src=DCAEVT2 with sync  dcbevt1src=DCBEVT1 with sync  dcbevt2src=DCBEVT2 with sync  pulsesel=Counter equals to zero (CTR=Zero)  blankinv=off  blankoffset=0  blankwidth=0  evsrcsel=Filtered version of DCAEVT1 (DCAEVT1FILT)  encape=off
  eQEP : c280xlib/eQEP  useModule=eQEP1  pcInputmode=Quadrature-count  externalClockrate=2x resolution: Count the rising/falling edge  swapPolarityselection=Counterclockwise  qdfOutputport=off  qapPolarityselection=on  qbpPolarityselection=on  qipPolarityselection=on  qspPolarityselection=off  igatePolarityselection=off  sampleTime=-1  pcOutputport=on  pcMaximumvalue=2^16-1  indexInitializationcheck=off  indexInitializationevent=Rising edge  strobeInitializationcheck=off  strobeInitializationevent=Rising edge  softwareInitializationcheck=off  softwareInitializationsource=Set to init value at start up  softwareInitializationmode=on  pcInitialvalue=2147483648  pcResetmode=Reset on the first index event  ieloutputport=on  indexEventlatch=Rising edge  seloutputport=off  strobeEventlatch=Rising edge  pcefOutputport=off  enableEqepcapture=off  qctmrOutputport=off  qcprdOutputport=off  captureTimerprescaler=128  upEventprescaler=128  overflowErrorflag=off  directionErrorflag=off  captureTimerposition=On position counter read  unitTimerperiod=100000000  captureTimerlatch=off  capturePeriodlatch=off  positionCounterlatch=off  soenPolarityselection=off  spselPolarityselection=Index pin is used for sync output  compareValuesource=Specify via dialog  shadowMode=Load on QPOSCNT=0  compareValue=4294967295  syncOutputwidth=1  polaritySyncoutput=Active high  watchdogEnable=off  watchdogTimer=65535  outport1Datatype=auto  outport2Datatype=auto  outport3Datatype=auto  outport4Datatype=auto  outport5Datatype=auto  outport6Datatype=auto  outport7Datatype=auto  outport8Datatype=auto  outport9Datatype=auto  outport10Datatype=auto  outport11Datatype=auto  outport12Datatype=auto  eqepinterrupt_pce=off  eqepinterrupt_qpe=off  eqepinterrupt_qdc=off  eqepinterrupt_wto=off  eqepinterrupt_pcu=off  eqepinterrupt_pco=off  eqepinterrupt_pcr=off  eqepinterrupt_pcm=off  eqepinterrupt_sel=off  eqepinterrupt_iel=off  eqepinterrupt_uto=off  pheOutputport=off  watchdogOutputport=off  outport13Datatype=auto  outport14Datatype=auto
  stop1 : Constant  Commented=on  Value=target.PWM_Counter_Period*0.5  OutDataTypeStr=uint16
  stop2 : Constant  Commented=on  Value=PWM_Counter_PeriodVel*0.5  OutDataTypeStr=uint16
  ThetaE : Outport
  speedfb : Outport  Port=2  VectorParamsAs1DForOutWhenUnconnected=off
  ThetaMec : Outport  Port=3
  wires:
  Speed Measurement/1 -> IIR Filter/1
  IndexFinder/1(EnClosedLoop) -> Data Store Write/1, Delay/1
  Quadrature Decoder/1 -> ThetaMec/1, Mechanical to Electrical Position/1, Speed Measurement/1
  Mechanical to Electrical Position/1 -> The/1
  eQEP/2 -> IndexFinder/1(In1), Quadrature Decoder/2
  NOT/1 -> IndexFinder/Enable
  eQEP/1 -> Quadrature Decoder/1
  Delay/1 -> NOT/1
  The/1 -> ThetaE/1
  stop1/1 -> ePWM8/1
  ADC_C2/1 -> Terminator/1
  IIR Filter/1 -> speedfb/1
  Constant1/1 -> Mechanical to Electrical Position/2

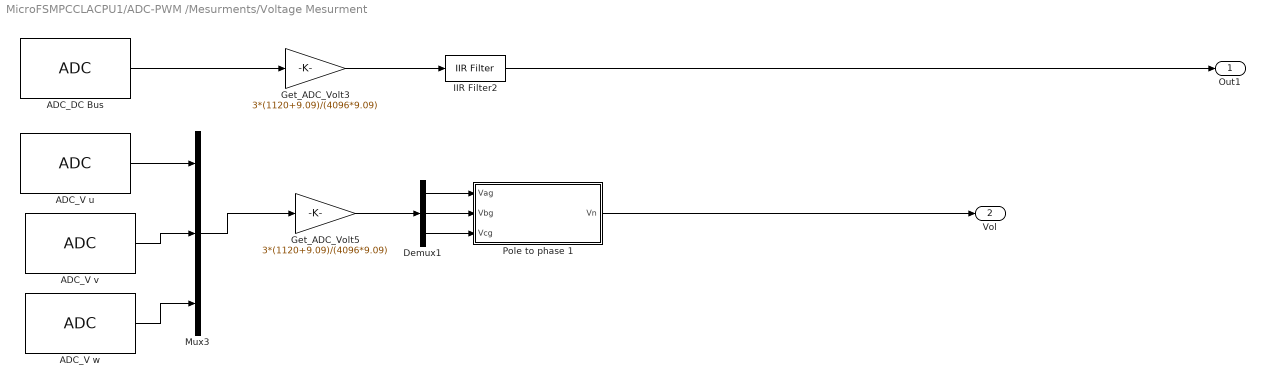
== system MicroFSMPCCLACPU1/ADC-PWM /Mesurments/Voltage Mesurment ==
  ADC_DC Bus : c2802xlib/ADC  blkParamProc=C2000_Type4  ADCModule=A  samplingMode=Single sample mode  ADCResolution=12-bit (Single-ended input)  useSOC1=SOC2  useSOC2=SOC0_SOC1  SOCAcquisitionWindow=15  SOCTriggerSource=ePWM1_ADCSOCA  SOCInterruptTrigger=No ADCINT  Ts=-1  dType=uint16  postInterrupt=off  interruptSel=ADCINT1  ADCINTContinuous=on  endma=off  chdma=1  conv1=ADCINA0  conv2=ADCINA0 and ADCINB0  conv1_Type4=ADCIN15  conv2_Type4=ADCIN0 and ADCIN1
  ADC_V u : c2802xlib/ADC  blkParamProc=C2000_Type4  ADCModule=D  samplingMode=Single sample mode  ADCResolution=12-bit (Single-ended input)  useSOC1=SOC0  useSOC2=SOC0_SOC1  SOCAcquisitionWindow=15  SOCTriggerSource=ePWM1_ADCSOCA  SOCInterruptTrigger=No ADCINT  Ts=-1  dType=uint16  postInterrupt=off  interruptSel=ADCINT1  ADCINTContinuous=on  endma=off  chdma=1  conv1=ADCINA0  conv2=ADCINA0 and ADCINB0  conv1_Type4=ADCIN1  conv2_Type4=ADCIN0 and ADCIN1
  ADC_V v : c2802xlib/ADC  blkParamProc=C2000_Type4  ADCModule=D  samplingMode=Single sample mode  ADCResolution=12-bit (Single-ended input)  useSOC1=SOC1  useSOC2=SOC0_SOC1  SOCAcquisitionWindow=15  SOCTriggerSource=ePWM1_ADCSOCA  SOCInterruptTrigger=No ADCINT  Ts=-1  dType=uint16  postInterrupt=off  interruptSel=ADCINT1  ADCINTContinuous=on  endma=off  chdma=1  conv1=ADCINA0  conv2=ADCINA0 and ADCINB0  conv1_Type4=ADCIN0  conv2_Type4=ADCIN0 and ADCIN1
  ADC_V w : c2802xlib/ADC  blkParamProc=C2000_Type4  ADCModule=B  samplingMode=Single sample mode  ADCResolution=12-bit (Single-ended input)  useSOC1=SOC2  useSOC2=SOC0_SOC1  SOCAcquisitionWindow=15  SOCTriggerSource=ePWM1_ADCSOCA  SOCInterruptTrigger=No ADCINT  Ts=-1  dType=uint16  postInterrupt=off  interruptSel=ADCINT1  ADCINTContinuous=on  endma=off  chdma=1  conv1=ADCINA0  conv2=ADCINA0 and ADCINB0  conv1_Type4=ADCIN4  conv2_Type4=ADCIN0 and ADCIN1
  Demux1 : Demux  Outputs=3
  Get_ADC_Volt3 : Gain  Gain=3*(1120+9.09)/(4096*9.09)  OutDataTypeStr=single  RndMeth=Simplest
  Get_ADC_Volt5 : Gain  Gain=3*(1120+9.09)/(4096*9.09)  OutDataTypeStr=single  RndMeth=Simplest
  IIR Filter2 : mcbcontrolslib/IIR Filter  VariantControl=Low Pass Filter  VariantSelect=Low-pass  FilterConstantInputType=Specify via dialog  Filter_constant=0.005  advancedSettings=off  Ts=10e-6  cutOff_freq=79.9774
  Mux3 : Mux  Inputs=3
  Pole to phase 1 : MATLAB Function  TreatAsAtomicUnit=on
  Out1 : Outport
  Vol : Outport  Port=2
  wires:
  ADC_V v/1 -> Mux3/2
  Mux3/1 -> Get_ADC_Volt5/1
  ADC_V u/1 -> Mux3/1
  Demux1/3 -> Pole to phase 1/3(Vcg)
  Demux1/2 -> Pole to phase 1/2(Vbg)
  Get_ADC_Volt5/1 -> Demux1/1
  Demux1/1 -> Pole to phase 1/1(Vag)
  IIR Filter2/1 -> Out1/1
  ADC_V w/1 -> Mux3/3
  Get_ADC_Volt3/1 -> IIR Filter2/1
  ADC_DC Bus/1 -> Get_ADC_Volt3/1
  Pole to phase 1/1(Vn) -> Vol/1

== system MicroFSMPCCLACPU1/PWM Module/Inverter (Code Generation)/Overcurrent protection ==
  In1 : Inport
  AND : Logic  IconShape=distinctive  AllPortsSameDT=off  OutDataTypeStr=boolean
  Digital Input : c2837xDlib/Digital Input  GPIO_Number=GPIO40~GPIO47  GPIO_Bit0=off  GPIO_Bit1=off  GPIO_Bit2=off  GPIO_Bit3=on  GPIO_Bit4=off  GPIO_Bit5=off  GPIO_Bit6=off  GPIO_Bit7=off  sampleTime=-1  dataType=boolean  GPIO_Bit0_Qualification=Sync to SYSCLKOUT  GPIO_Bit1_Qualification=Sync to SYSCLKOUT  GPIO_Bit2_Qualification=Sync to SYSCLKOUT  GPIO_Bit3_Qualification=Sync to SYSCLKOUT  GPIO_Bit4_Qualification=Sync to SYSCLKOUT  GPIO_Bit5_Qualification=Sync to SYSCLKOUT  GPIO_Bit6_Qualification=Sync to SYSCLKOUT  GPIO_Bit7_Qualification=Sync to SYSCLKOUT  Qualification_Period=-1
  Digital Output1 : c2837xDlib/Digital Output  GPIO_Number=GPIO24~GPIO31  GPIO_Bit0=off  GPIO_BIT0_Toggle=on  GPIO_Bit1=off  GPIO_BIT1_Toggle=off  GPIO_Bit2=off  GPIO_BIT2_Toggle=off  GPIO_Bit3=off  GPIO_BIT3_Toggle=off  GPIO_Bit4=off  GPIO_BIT4_Toggle=off  GPIO_Bit5=off  GPIO_BIT5_Toggle=off  GPIO_Bit6=off  GPIO_BIT6_Toggle=off  GPIO_Bit7=on  GPIO_BIT7_Toggle=off
  Digital Output2 : c2837xDlib/Digital Output  GPIO_Number=GPIO8~GPIO15  GPIO_Bit0=off  GPIO_BIT0_Toggle=on  GPIO_Bit1=on  GPIO_BIT1_Toggle=off  GPIO_Bit2=off  GPIO_BIT2_Toggle=off  GPIO_Bit3=off  GPIO_BIT3_Toggle=off  GPIO_Bit4=off  GPIO_BIT4_Toggle=off  GPIO_Bit5=off  GPIO_BIT5_Toggle=off  GPIO_Bit6=off  GPIO_BIT6_Toggle=off  GPIO_Bit7=off  GPIO_BIT7_Toggle=off
  Enable1 : DataStoreRead  DataStoreName=EnClosedLoop  IndexOptions=Index vector (dialog)  Indices=1  OutputSizes=1
  NOT : Logic  Operator=NOT  IconShape=distinctive  AllPortsSameDT=off  OutDataTypeStr=boolean
  ata Type Conversion1 : DataTypeConversion  OutDataTypeStr=dataType  SaturateOnIntegerOverflow=off  RndMeth=Floor
  Out1 : Outport
  wires:
  NOT/1 -> AND/2, Digital Output1/1
  Digital Input/1 -> NOT/1  "PWM_Enable"
  AND/1 -> Out1/1
  In1/1 -> AND/1
  ata Type Conversion1/1 -> Digital Output2/1
  Enable1/1 -> ata Type Conversion1/1

== system MicroFSMPCCLACPU1/ADC-PWM /Control_System/CLA Subsystem Current control/Clark Transform1 ==
  Fcem : Inport
  Iabc : Inport  Port=2
  Clarke Transform1 : mcbcontrolslib/Clarke Transform  VariantControl=Variant2  PhaseInput=Two inputs  EnPowerInv=off
  Clarke Transform2 : eeTransforms/Clarke Transform  Commented=on  PowerInvariant=off
  Demux : Demux  Outputs=3
  Demux1 : Demux  Commented=on  Outputs=3
  Mux1 : Mux  Commented=on  Inputs=2
  Mux3 : Mux  Inputs=2
  Terminator1 : Terminator  Commented=on
  Iab : Outport
  Fcemab : Outport  Port=2
  wires:
  Demux1/1 -> Mux1/1
  Fcem/1 -> Clarke Transform2/1
  Demux1/2 -> Mux1/2
  Mux3/1 -> Iab/1
  Clarke Transform2/1 -> Demux1/1
  Mux1/1 -> Fcemab/1
  Demux1/3 -> Terminator1/1
  Demux/1 -> Clarke Transform1/1
  Demux/2 -> Clarke Transform1/2
  Iabc/1 -> Demux/1
  Clarke Transform1/1 -> Mux3/1
  Clarke Transform1/2 -> Mux3/2

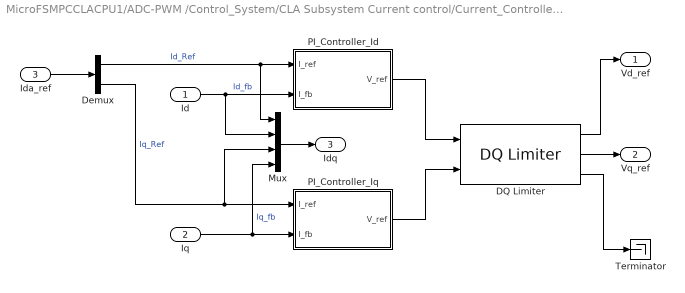
== system MicroFSMPCCLACPU1/ADC-PWM /Control_System/CLA Subsystem Current control/Current_Controllers ==
  Id : Inport
  Iq : Inport  Port=2
  Ida_ref : Inport  Port=3
  DQ Limiter : mcbcontrolslib/DQ Limiter  satMethodInputType=Specify via dialog  satMethodSelected=D-Q equivalence  satLimitInputType=Specify via dialog  Vmax=inverter.V_dc/sqrt(3) *0.95
  Demux : Demux  Outputs=2
  Mux : Mux
  PI_Controller_Id : Subsystem
  PI_Controller_Iq : Subsystem
  Terminator : Terminator
  Vd_ref : Outport  VectorParamsAs1DForOutWhenUnconnected=off
  Vq_ref : Outport  Port=2  VectorParamsAs1DForOutWhenUnconnected=off
  Idq : Outport  Port=3  VectorParamsAs1DForOutWhenUnconnected=off
  wires:
  Iq/1 -> Mux/4, PI_Controller_Iq/2(I_fb)  "Iq_fb"
  Id/1 -> Mux/2, PI_Controller_Id/2(I_fb)  "Id_fb"
  Demux/1 -> Mux/1, PI_Controller_Id/1(I_ref)  "Id_Ref"
  Demux/2 -> Mux/3, PI_Controller_Iq/1(I_ref)  "Iq_Ref"
  Ida_ref/1 -> Demux/1
  Mux/1 -> Idq/1
  PI_Controller_Id/1(V_ref) -> DQ Limiter/1
  PI_Controller_Iq/1(V_ref) -> DQ Limiter/2
  DQ Limiter/2 -> Vq_ref/1
  DQ Limiter/1 -> Vd_ref/1
  DQ Limiter/3 -> Terminator/1

== system MicroFSMPCCLACPU1/ADC-PWM /Control_System/CLA Subsystem Current control/Subsystem ==
  FCEM : Inport
  Demux5 : Demux  Outputs=2
  IIR Filter10 : mcbcontrolslib/IIR Filter  VariantControl=Low Pass Filter  VariantSelect=Low-pass  Filter_constant=0.2  advancedSettings=off  Ts=5e-5  cutOff_freq=795.7747
  IIR Filter9 : mcbcontrolslib/IIR Filter  VariantControl=Low Pass Filter  VariantSelect=Low-pass  Filter_constant=0.2  advancedSettings=off  Ts=5e-5  cutOff_freq=795.7747
  Mux7 : Mux  Inputs=2
  Out1 : Outport
  wires:
  IIR Filter9/1 -> Mux7/1
  Demux5/1 -> IIR Filter9/1
  Demux5/2 -> IIR Filter10/1
  IIR Filter10/1 -> Mux7/2
  Mux7/1 -> Out1/1
  FCEM/1 -> Demux5/1

== system MicroFSMPCCLACPU1/ADC-PWM /Control_System/Clark Transform Filter/Clarke Transformation ==
  Ia : Inport
  Ib : Inport  Port=2
  1 : Constant  Value=0.57735026918963  OutDataTypeStr=single
  2 : Constant  Value=2  OutDataTypeStr=single  SampleTime=Inf
  Product : Product  OutDataTypeStr=single
  Product1 : Product  OutDataTypeStr=Inherit: Same as first input
  Sum1 : Sum  Inputs=|++  OutDataTypeStr=Inherit: Same as first input
  Out1 : Outport
  Out2 : Outport  Port=2
  wires:
  Ib/1 -> Product/2
  Ia/1 -> Out1/1, Sum1/1
  Sum1/1 -> Product1/2
  2/1 -> Product/1
  Product1/1 -> Out2/1
  Product/1 -> Sum1/2
  1/1 -> Product1/1

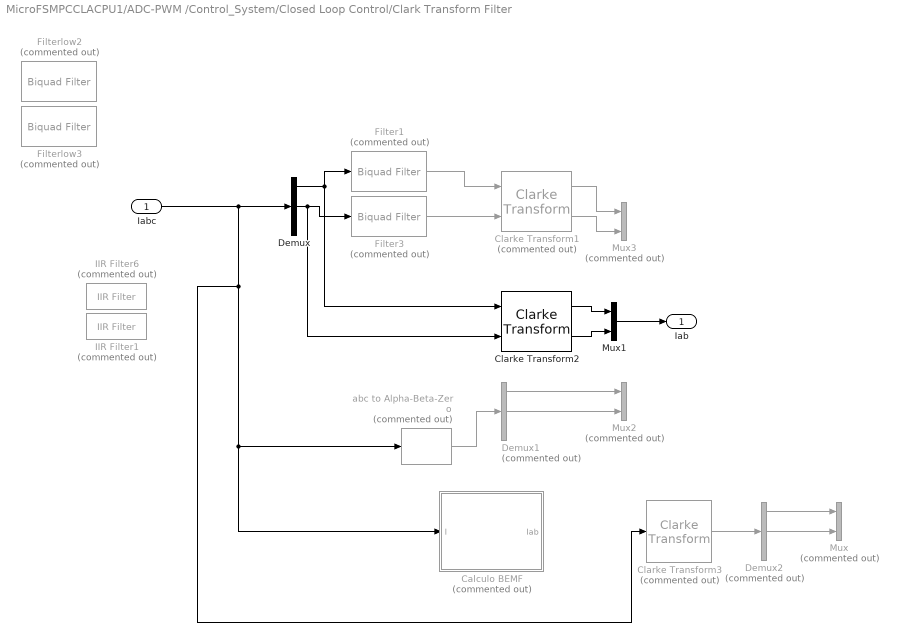
== system MicroFSMPCCLACPU1/ADC-PWM /Control_System/Closed Loop Control/Clark Transform Filter ==
  Iabc : Inport
  Calculo BEMF : MATLAB Function  Commented=on  TreatAsAtomicUnit=on
  Clarke Transform1 : mcbcontrolslib/Clarke Transform  Commented=on  VariantControl=Variant2  PhaseInput=Two inputs  EnPowerInv=off
  Clarke Transform2 : mcbcontrolslib/Clarke Transform  VariantControl=Variant2  PhaseInput=Two inputs  EnPowerInv=off
  Clarke Transform3 : eeTransforms/Clarke Transform  Commented=on  PowerInvariant=off
  Demux : Demux  Outputs=3
  Demux1 : Demux  Commented=on  Outputs=3
  Demux2 : Demux  Commented=on  Outputs=3
  Filter1 : dsparch4/Biquad Filter  Tag=BlockMethodSubSystem  Commented=on  FilterSource=Dialog parameters  CoeffSource=Specify via dialog  FilterObject=BQF  IIRFiltStruct=Direct form II  BiQuadCoeffs=[1 -1.98875017224897266 1 1 -1.91515179130977486 0.931749383715403057;1 -1.99505427791452594 1 1 -1.96656906751029581 0.969754532157833138;1 -1.98427320030682486 1 1 -1.976612836271463 0.993613655100407445;1 -1.99646490719288527 1 1 -1.99394420928600846 0.997198518109316367]  ScaleValues=[2.08022492851452157;2.08022492851452157;0.454207780323216626;0.454207780323216626;1]  IC=0  ICnum=0  ICden=0  a0Flag=Warning  optimizeScaleValues=on  ScaleValueMode=Specify via input port (g)  InputProcessing=Columns as channels (frame based)  roundingMode=Floor  overflowMode=off  scaleValueFracLength=14  denProdOutputFracLength=30  denAccumFracLength=30  secondMemoryFracLength=15
  Filter3 : dsparch4/Biquad Filter  Tag=BlockMethodSubSystem  Commented=on  FilterSource=Dialog parameters  CoeffSource=Specify via dialog  FilterObject=BQF  IIRFiltStruct=Direct form II  BiQuadCoeffs=[1 -1.98875017224897266 1 1 -1.91515179130977486 0.931749383715403057;1 -1.99505427791452594 1 1 -1.96656906751029581 0.969754532157833138;1 -1.98427320030682486 1 1 -1.976612836271463 0.993613655100407445;1 -1.99646490719288527 1 1 -1.99394420928600846 0.997198518109316367]  ScaleValues=[2.08022492851452157;2.08022492851452157;0.454207780323216626;0.454207780323216626;1]  IC=0  ICnum=0  ICden=0  a0Flag=Warning  optimizeScaleValues=on  ScaleValueMode=Specify via input port (g)  InputProcessing=Columns as channels (frame based)  roundingMode=Floor  overflowMode=off  scaleValueFracLength=14  denProdOutputFracLength=30  denAccumFracLength=30  secondMemoryFracLength=15
  Filterlow2 : dsparch4/Biquad Filter  Tag=BlockMethodSubSystem  Commented=on  FilterSource=Dialog parameters  CoeffSource=Specify via dialog  FilterObject=BQF  IIRFiltStruct=Direct form II  BiQuadCoeffs=[1 -1.97442720001352012 1 1 -1.88787110810661729 0.896562526404252491;1 -1.99220105321702157 1 1 -1.98338455309476136 0.99034176901857085]  ScaleValues=[0.843607290826595912;0.355280663387145257;1]  IC=0  ICnum=0  ICden=0  a0Flag=Warning  optimizeScaleValues=on  ScaleValueMode=Specify via input port (g)  InputProcessing=Columns as channels (frame based)  roundingMode=Floor  overflowMode=off  scaleValueFracLength=14  denProdOutputFracLength=30  denAccumFracLength=30  secondMemoryFracLength=15
  Filterlow3 : dsparch4/Biquad Filter  Tag=BlockMethodSubSystem  Commented=on  FilterSource=Dialog parameters  CoeffSource=Specify via dialog  FilterObject=BQF  IIRFiltStruct=Direct form II  BiQuadCoeffs=[1 -1.97442720001352012 1 1 -1.88787110810661729 0.896562526404252491;1 -1.99220105321702157 1 1 -1.98338455309476136 0.99034176901857085]  ScaleValues=[0.843607290826595912;0.355280663387145257;1]  IC=0  ICnum=0  ICden=0  a0Flag=Warning  optimizeScaleValues=on  ScaleValueMode=Specify via input port (g)  InputProcessing=Columns as channels (frame based)  roundingMode=Floor  overflowMode=off  scaleValueFracLength=14  denProdOutputFracLength=30  denAccumFracLength=30  secondMemoryFracLength=15
  IIR Filter1 : mcbcontrolslib/IIR Filter  Commented=on  VariantControl=Low Pass Filter  VariantSelect=Low-pass  Filter_constant=0.3  advancedSettings=off  Ts=5e-5  cutOff_freq=1364.1852
  IIR Filter6 : mcbcontrolslib/IIR Filter  Commented=on  VariantControl=Low Pass Filter  VariantSelect=Low-pass  Filter_constant=0.3  advancedSettings=off  Ts=5e-5  cutOff_freq=1364.1852
  Mux : Mux  Commented=on  Inputs=2
  Mux1 : Mux  Inputs=2
  Mux2 : Mux  Commented=on  Inputs=2
  Mux3 : Mux  Commented=on  Inputs=2
  abc to Alpha-Beta-Zero : spsabctoAlphaBetaZeroLib/abc to Alpha-Beta-Zero  Commented=on
  Iab : Outport
  wires:
  Iabc/1 -> Clarke Transform3/1, Calculo BEMF/1(I), abc to Alpha-Beta-Zero/1, Demux/1
  Clarke Transform1/1 -> Mux3/1
  Clarke Transform1/2 -> Mux3/2
  Filter3/1 -> Clarke Transform1/2
  Filter1/1 -> Clarke Transform1/1
  Clarke Transform2/1 -> Mux1/1
  Clarke Transform2/2 -> Mux1/2
  Demux/2 -> Clarke Transform2/2, Filter3/1
  Demux/1 -> Filter1/1, Clarke Transform2/1
  abc to Alpha-Beta-Zero/1 -> Demux1/1
  Demux1/1 -> Mux2/1
  Demux1/2 -> Mux2/2
  Clarke Transform3/1 -> Demux2/1
  Demux2/1 -> Mux/1
  Demux2/2 -> Mux/2
  Mux1/1 -> Iab/1

== system MicroFSMPCCLACPU1/ADC-PWM /Control_System/Closed Loop Control/Clark Transform1 ==
  Fcem : Inport
  Iabc : Inport  Port=2
  Clarke Transform1 : mcbcontrolslib/Clarke Transform  VariantControl=Variant2  PhaseInput=Two inputs  EnPowerInv=off
  Clarke Transform2 : eeTransforms/Clarke Transform  Commented=on  PowerInvariant=off
  Demux : Demux  Outputs=3
  Demux1 : Demux  Commented=on  Outputs=3
  Mux1 : Mux  Commented=on  Inputs=2
  Mux3 : Mux  Inputs=2
  Terminator1 : Terminator  Commented=on
  Iab : Outport
  Fcemab : Outport  Port=2
  wires:
  Demux1/1 -> Mux1/1
  Fcem/1 -> Clarke Transform2/1
  Demux1/2 -> Mux1/2
  Mux3/1 -> Iab/1
  Clarke Transform2/1 -> Demux1/1
  Mux1/1 -> Fcemab/1
  Demux1/3 -> Terminator1/1
  Demux/1 -> Clarke Transform1/1
  Demux/2 -> Clarke Transform1/2
  Iabc/1 -> Demux/1
  Clarke Transform1/1 -> Mux3/1
  Clarke Transform1/2 -> Mux3/2
